simulink model "lab3"  (R2017b)
settings: Solver=ode45  StartTime=0.0  StopTime=100  MaxStep=0.1  RelTol=1e-3
libraries: simulink x2
settings Model: Creator=niquit  LastModifiedBy=niquit

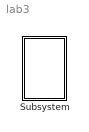
== system lab3 ==
  Subsystem : Subsystem  mask{g=9.81, m=2, l=2, k=5, r0=3, r1=1, fi0=0.1, fi1=0.1}

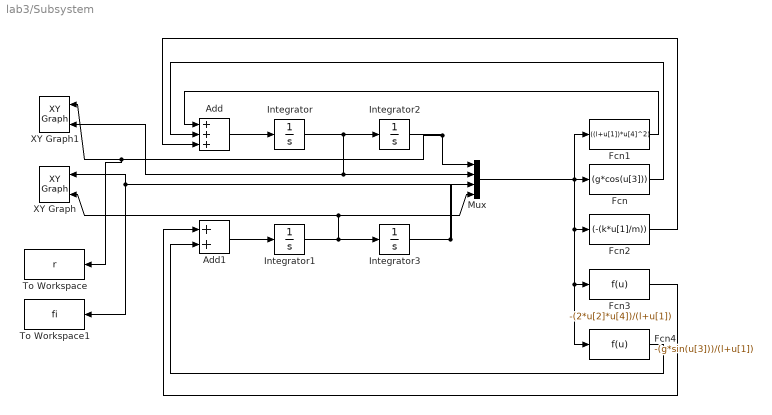
== system lab3/Subsystem ==
  Add : Sum  Inputs=+++
  Add1 : Sum
  Fcn : Fcn  Expr=(g*cos(u[3]))
  Fcn1 : Fcn  Expr=((l+u[1])*u[4]^2)
  Fcn2 : Fcn  Expr=(-(k*u[1]/m))
  Fcn3 : Fcn  Expr=-(2*u[2]*u[4])/(l+u[1])
  Fcn4 : Fcn  Expr=-(g*sin(u[3]))/(l+u[1])
  Integrator : Integrator  InitialCondition=r1
  Integrator1 : Integrator  InitialCondition=fi1
  Integrator2 : Integrator  InitialCondition=r0
  Integrator3 : Integrator  InitialCondition=fi0
  Mux : Mux
  To Workspace : ToWorkspace  VariableName=r  SampleTime=-1
  To Workspace1 : ToWorkspace  VariableName=fi  SampleTime=-1
  XY Graph : simulink/Sinks/XY Graph  xmin=-0.2  xmax=0.2  ymin=-0.2  ymax=0.2  st=-1
  XY Graph1 : simulink/Sinks/XY Graph  xmin=2.5  xmax=5.5  ymin=-2  ymax=2  st=-1
  wires:
  Add/1 -> Integrator/1
  Add1/1 -> Integrator1/1
  Fcn2/1 -> Add/3
  Integrator2/1 -> To Workspace/1, XY Graph1/1, Mux/1
  Integrator/1 -> Mux/2, XY Graph1/2, Integrator2/1
  Integrator1/1 -> XY Graph/2, Mux/4, Integrator3/1
  Mux/1 -> Fcn4/1, Fcn3/1, Fcn2/1, Fcn/1, Fcn1/1
  Fcn1/1 -> Add/1
  Fcn/1 -> Add/2
  Fcn4/1 -> Add1/2
  Fcn3/1 -> Add1/1
  Integrator3/1 -> To Workspace1/1, XY Graph/1, Mux/3
